simulink model "Bidir3"  (R2024a)
settings: Solver=VariableStepAuto  StartTime=0.0  StopTime=70  MaxStep=0.1  RelTol=1e-3
libraries: simulink x10
settings Model: Creator=SEPTPFNK  LastModifiedBy=skoge
settings DataIOCC: SaveFormat=Array  SaveOutput=off  DSMLogging=off  ReturnWorkspaceOutputs=off  TimeSaveName=t
settings OptimizationCC: ReuseModelBlockBuffer=off
settings RTWCC: GPUComputeCapability=3.5

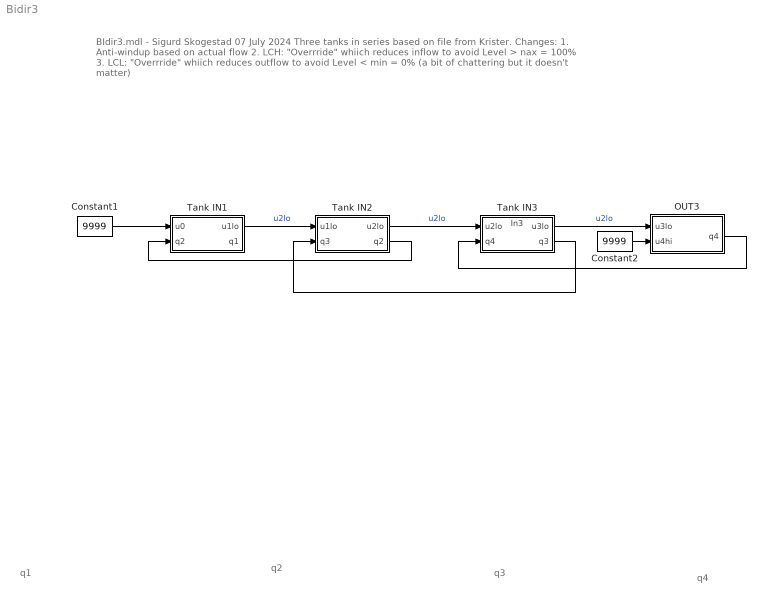
== system Bidir3 ==
  note: q1
  note: BIdir3.mdl - Sigurd Skogestad 07 July 2024
      | Three tanks in series based on file from Krister.
      |
      | Changes: 1. Anti-windup based on actual flow
      | 2. LCH: "Overrride" whiich reduces inflow to avoid Level > nax = 100%
      | 3. LCL: "Overrride" whiich reduces outflow to avoid Level < min = 0% (a bit of chattering but it doesn't matter)
  note: q2
  note: q3
  note: q4
  Constant1 : Constant  Value=9999
  Constant2 : Constant  Value=9999
  OUT3 : Subsystem
  Tank IN1 : Subsystem
  Tank IN2 : Subsystem
  Tank IN3 : Subsystem
      settings: PortSchema="{\"entries\":[{\"content\":{\"sides\":[{\"content\":{\"connectorIds\":[\"In1\",\"In2\"]},\"type\":\"ConnectorPlacement.EquallySpacedRectSide\",\"uuid\":\"ff44d203-131c-4583-b6b4-863d22efac0d\"},{\"content\":{\"connectorIds\":[\"Out1\",\"Out2\"],\"side\":\"RIGHT\"},\"type\":\"ConnectorPlacement.EquallySpacedRectSide\",\"uuid\":\"9e6c79fa-f849-4fea-b46c-ba618541df73\"},{\"content\":{\"connectorIds\":[\"In3\"],\"side\":\"TOP\"},\"type\":\"ConnectorPlacement.EquallySpacedRectSide\",\"uuid\":\"7639274b-f52c-4ba2-a8a4-a7eece00f8f0\"}]},\"type\":\"ConnectorPlacement.EquallySpacedConnector\",\"uuid\":\"d074d2e5-96ed-48a1-ad28-1a607b55dcd0\"}],\"packageUris\":[\"http://schema.mathworks.com/mf0/Connector/R2020b\"],\"version\":\"1.0\"}"
  wires:
  Tank IN1/1(u1lo) -> Tank IN2/1(u1lo)  "u2lo"
  Tank IN2/2(q2) -> Tank IN1/2(q2)
  Constant1/1 -> Tank IN1/1(u0)
  Tank IN2/1(u2lo) -> Tank IN3/1(u2lo)  "u2lo"
  Tank IN3/2(q3) -> Tank IN2/2(q3)
  Tank IN3/1(u3lo) -> OUT3/1(u3lo)  "u2lo"
  Constant2/1 -> OUT3/2(u4hi)
  OUT3/1(q4) -> Tank IN3/2(q4)

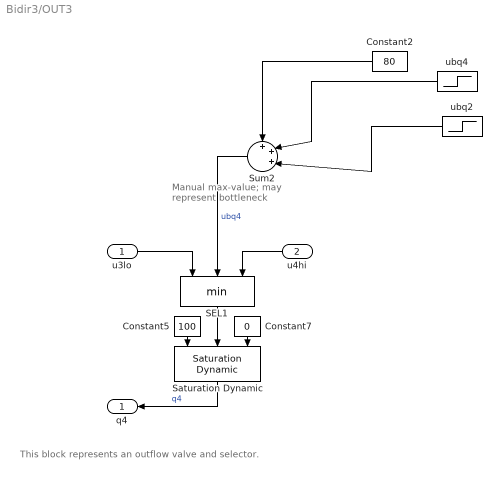
== system Bidir3/OUT3 ==
  note: This block represents an outflow valve and selector.
  note: Manual max-value; may represent bottleneck
  u3lo : Inport
  u4hi : Inport  Port=2
  Constant2 : Constant  Value=80
  Constant5 : Constant  Value=100
  Constant7 : Constant  Value=0
  SEL1 : MinMax  Inputs=3
  Saturation Dynamic : simulink/Discontinuities/Saturation Dynamic  OutMin=[]  OutMax=[]  OutDataTypeStr=Inherit: Same as second input  OutDataType=fixdt(1, 16)  OutScaling=2^-10  DoSatur=off
  Sum2 : Sum  Inputs=+++|
  ubq2 : Step  Time=20  After=-50  SampleTime=0
  ubq4 : Step  Time=10  After=10  SampleTime=0
  q4 : Outport
  wires:
  u3lo/1 -> SEL1/1
  SEL1/1 -> Saturation Dynamic/2
  Constant5/1 -> Saturation Dynamic/1
  Constant7/1 -> Saturation Dynamic/3
  Sum2/1 -> SEL1/2  "ubq4"
  Constant2/1 -> Sum2/1
  ubq2/1 -> Sum2/3
  ubq4/1 -> Sum2/2
  Saturation Dynamic/1 -> q4/1  "q4"
  u4hi/1 -> SEL1/3

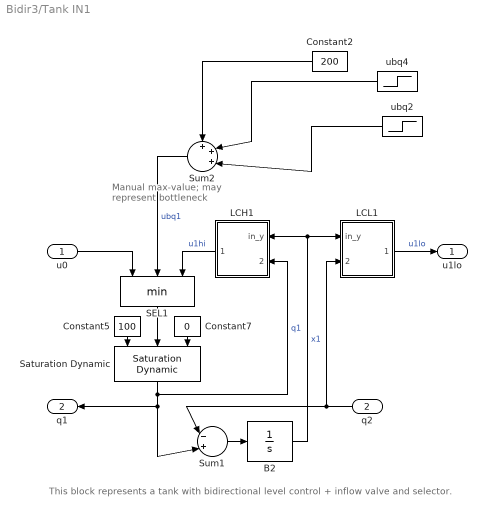
== system Bidir3/Tank IN1 ==
  note: This block represents a tank with bidirectional level control + inflow valve and selector.
  note: Manual max-value; may represent bottleneck
  u0 : Inport
  q2 : Inport  Port=2
  B2 : Integrator  InitialCondition=80  LimitOutput=on  UpperSaturationLimit=200  LowerSaturationLimit=-100
  Constant2 : Constant  Value=200
  Constant5 : Constant  Value=100
  Constant7 : Constant  Value=0
  LCH1 : Subsystem  mask(PID-controller){Kc=1, Ti=4, Tarw=2, r0=80, u0=80, yMin=0, yMax=100, uMin=0, uMax=100}
      mask prompts: Tarw "T_arw"; r0 "Setpoint:"; u0 "Initial output:"
      mask help: PID-controller
      mask Help:
      | <P> PID-controller with beta-factor, limiting, ARW etc </P>
      | 
      | Inputs: <P>
      |  <UL>
      |   1 = r (setpoint) <BR>
      |   2 = y (process value) <BR>
      |   3  = u0 (control signal offset) <BR>
      |  </UL>
      |  </P>
      | Outputs: <P>
      |  <UL>
      |    1 = u (control signal) <BR>
      |    2 = Proportional part  <BR>
      |    3 = Integral part  <BR>
      |    4 = Derivative part  <BR>
      |    5 = raw signal, without ARW  <BR>
      |  </UL>
      |  </P>
      mask Display:
      | disp(['PI' 10 10 10])
      | port_label('input',1,'y')
      | port_label('input',2,'uaw')
      | port_label('output',1,'u')
  LCL1 : Subsystem  mask(PID-controller){Kc=-1, Ti=4, Tarw=2, r0=10, u0=80, yMin=0, yMax=100, uMin=0, uMax=100}
      mask prompts: Tarw "T_arw"; r0 "Setpoint:"; u0 "Initial output:"
      mask help: PID-controller
      mask Help:
      | <P> PID-controller with beta-factor, limiting, ARW etc </P>
      | 
      | Inputs: <P>
      |  <UL>
      |   1 = r (setpoint) <BR>
      |   2 = y (process value) <BR>
      |   3  = u0 (control signal offset) <BR>
      |  </UL>
      |  </P>
      | Outputs: <P>
      |  <UL>
      |    1 = u (control signal) <BR>
      |    2 = Proportional part  <BR>
      |    3 = Integral part  <BR>
      |    4 = Derivative part  <BR>
      |    5 = raw signal, without ARW  <BR>
      |  </UL>
      |  </P>
      mask Display:
      | disp(['PI' 10 10 10])
      | port_label('input',1,'y')
      | port_label('input',2,'uaw')
      | port_label('output',1,'u')
  SEL1 : MinMax  Inputs=3
  Saturation Dynamic : simulink/Discontinuities/Saturation Dynamic  OutMin=[]  OutMax=[]  OutDataTypeStr=Inherit: Same as second input  OutDataType=fixdt(1, 16)  OutScaling=2^-10  DoSatur=off
  Sum1 : Sum  Inputs=|-+|
  Sum2 : Sum  Inputs=+++|
  ubq2 : Step  Time=60  After=-20  SampleTime=0
  ubq4 : Step  Time=40  After=-170  SampleTime=0
  u1lo : Outport
  q1 : Outport  Port=2
  wires:
  B2/1 -> LCL1/1(in_y), LCH1/1(in_y)  "x1"
  u0/1 -> SEL1/1
  SEL1/1 -> Saturation Dynamic/2
  Constant5/1 -> Saturation Dynamic/1
  LCH1/1(out_u) -> SEL1/3  "u1hi"
  Sum1/1 -> B2/1
  Constant7/1 -> Saturation Dynamic/3
  Saturation Dynamic/1 -> Sum1/2, q1/1, LCH1/2(in_yaw)  "q1"
  q2/1 -> LCL1/2(in_yaw), Sum1/1
  Sum2/1 -> SEL1/2  "ubq1"
  Constant2/1 -> Sum2/1
  ubq2/1 -> Sum2/3
  ubq4/1 -> Sum2/2
  LCL1/1(out_u) -> u1lo/1  "u1lo"

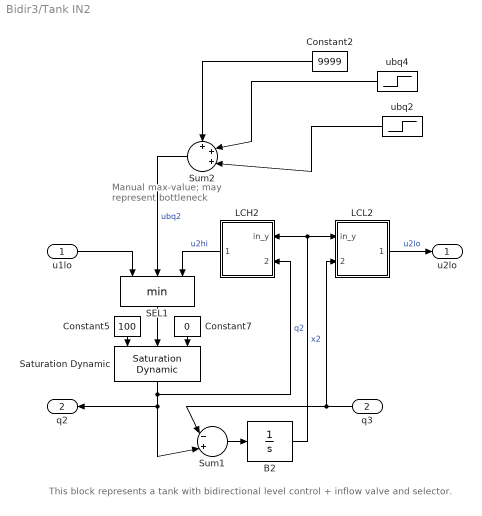
== system Bidir3/Tank IN2 ==
  note: This block represents a tank with bidirectional level control + inflow valve and selector.
  note: Manual max-value; may represent bottleneck
  u1lo : Inport
  q3 : Inport  Port=2
  B2 : Integrator  InitialCondition=80  LimitOutput=on  UpperSaturationLimit=200  LowerSaturationLimit=-100
  Constant2 : Constant  Value=9999
  Constant5 : Constant  Value=100
  Constant7 : Constant  Value=0
  LCH2 : Subsystem  mask(PID-controller){Kc=1, Ti=4, Tarw=2, r0=80, u0=80, yMin=0, yMax=100, uMin=0, uMax=100}
      mask prompts: Tarw "T_arw"; r0 "Setpoint:"; u0 "Initial output:"
      mask help: PID-controller
      mask Help:
      | <P> PID-controller with beta-factor, limiting, ARW etc </P>
      | 
      | Inputs: <P>
      |  <UL>
      |   1 = r (setpoint) <BR>
      |   2 = y (process value) <BR>
      |   3  = u0 (control signal offset) <BR>
      |  </UL>
      |  </P>
      | Outputs: <P>
      |  <UL>
      |    1 = u (control signal) <BR>
      |    2 = Proportional part  <BR>
      |    3 = Integral part  <BR>
      |    4 = Derivative part  <BR>
      |    5 = raw signal, without ARW  <BR>
      |  </UL>
      |  </P>
      mask Display:
      | disp(['PI' 10 10 10])
      | port_label('input',1,'y')
      | port_label('input',2,'uaw')
      | port_label('output',1,'u')
  LCL2 : Subsystem  mask(PID-controller){Kc=-1, Ti=4, Tarw=2, r0=10, u0=80, yMin=0, yMax=100, uMin=0, uMax=100}
      mask prompts: Tarw "T_arw"; r0 "Setpoint:"; u0 "Initial output:"
      mask help: PID-controller
      mask Help:
      | <P> PID-controller with beta-factor, limiting, ARW etc </P>
      | 
      | Inputs: <P>
      |  <UL>
      |   1 = r (setpoint) <BR>
      |   2 = y (process value) <BR>
      |   3  = u0 (control signal offset) <BR>
      |  </UL>
      |  </P>
      | Outputs: <P>
      |  <UL>
      |    1 = u (control signal) <BR>
      |    2 = Proportional part  <BR>
      |    3 = Integral part  <BR>
      |    4 = Derivative part  <BR>
      |    5 = raw signal, without ARW  <BR>
      |  </UL>
      |  </P>
      mask Display:
      | disp(['PI' 10 10 10])
      | port_label('input',1,'y')
      | port_label('input',2,'uaw')
      | port_label('output',1,'u')
  SEL1 : MinMax  Inputs=3
  Saturation Dynamic : simulink/Discontinuities/Saturation Dynamic  OutMin=[]  OutMax=[]  OutDataTypeStr=Inherit: Same as second input  OutDataType=fixdt(1, 16)  OutScaling=2^-10  DoSatur=off
  Sum1 : Sum  Inputs=|-+|
  Sum2 : Sum  Inputs=+++|
  ubq2 : Step  Time=20  After=-20  SampleTime=0
  ubq4 : Step  Time=2  After=20  SampleTime=0
  u2lo : Outport
  q2 : Outport  Port=2
  wires:
  B2/1 -> LCL2/1(in_y), LCH2/1(in_y)  "x2"
  u1lo/1 -> SEL1/1
  SEL1/1 -> Saturation Dynamic/2
  Constant5/1 -> Saturation Dynamic/1
  LCH2/1(out_u) -> SEL1/3  "u2hi"
  Sum1/1 -> B2/1
  Constant7/1 -> Saturation Dynamic/3
  Saturation Dynamic/1 -> LCH2/2(in_yaw), Sum1/2, q2/1  "q2"
  q3/1 -> LCL2/2(in_yaw), Sum1/1
  Sum2/1 -> SEL1/2  "ubq2"
  Constant2/1 -> Sum2/1
  ubq2/1 -> Sum2/3
  ubq4/1 -> Sum2/2
  LCL2/1(out_u) -> u2lo/1  "u2lo"

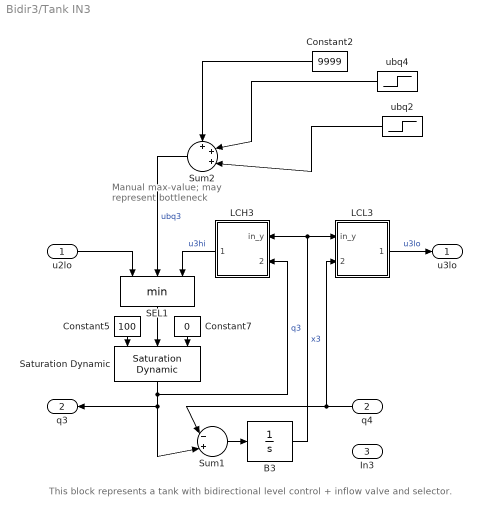
== system Bidir3/Tank IN3 ==
  note: This block represents a tank with bidirectional level control + inflow valve and selector.
  note: Manual max-value; may represent bottleneck
  u2lo : Inport
  q4 : Inport  Port=2
  In3 : Inport  Port=3
  B3 : Integrator  InitialCondition=80  LimitOutput=on  UpperSaturationLimit=200  LowerSaturationLimit=-100
  Constant2 : Constant  Value=9999
  Constant5 : Constant  Value=100
  Constant7 : Constant  Value=0
  LCH3 : Subsystem  mask(PID-controller){Kc=1, Ti=4, Tarw=2, r0=80, u0=80, yMin=0, yMax=100, uMin=0, uMax=100}
      mask prompts: Tarw "T_arw"; r0 "Setpoint:"; u0 "Initial output:"
      mask help: PID-controller
      mask Help:
      | <P> PID-controller with beta-factor, limiting, ARW etc </P>
      | 
      | Inputs: <P>
      |  <UL>
      |   1 = r (setpoint) <BR>
      |   2 = y (process value) <BR>
      |   3  = u0 (control signal offset) <BR>
      |  </UL>
      |  </P>
      | Outputs: <P>
      |  <UL>
      |    1 = u (control signal) <BR>
      |    2 = Proportional part  <BR>
      |    3 = Integral part  <BR>
      |    4 = Derivative part  <BR>
      |    5 = raw signal, without ARW  <BR>
      |  </UL>
      |  </P>
      mask Display:
      | disp(['PI' 10 10 10])
      | port_label('input',1,'y')
      | port_label('input',2,'uaw')
      | port_label('output',1,'u')
  LCL3 : Subsystem  mask(PID-controller){Kc=-1, Ti=4, Tarw=2, r0=10, u0=80, yMin=0, yMax=100, uMin=0, uMax=100}
      mask prompts: Tarw "T_arw"; r0 "Setpoint:"; u0 "Initial output:"
      mask help: PID-controller
      mask Help:
      | <P> PID-controller with beta-factor, limiting, ARW etc </P>
      | 
      | Inputs: <P>
      |  <UL>
      |   1 = r (setpoint) <BR>
      |   2 = y (process value) <BR>
      |   3  = u0 (control signal offset) <BR>
      |  </UL>
      |  </P>
      | Outputs: <P>
      |  <UL>
      |    1 = u (control signal) <BR>
      |    2 = Proportional part  <BR>
      |    3 = Integral part  <BR>
      |    4 = Derivative part  <BR>
      |    5 = raw signal, without ARW  <BR>
      |  </UL>
      |  </P>
      mask Display:
      | disp(['PI' 10 10 10])
      | port_label('input',1,'y')
      | port_label('input',2,'uaw')
      | port_label('output',1,'u')
  SEL1 : MinMax  Inputs=3
  Saturation Dynamic : simulink/Discontinuities/Saturation Dynamic  OutMin=[]  OutMax=[]  OutDataTypeStr=Inherit: Same as second input  OutDataType=fixdt(1, 16)  OutScaling=2^-10  DoSatur=off
  Sum1 : Sum  Inputs=|-+|
  Sum2 : Sum  Inputs=+++|
  ubq2 : Step  Time=20  After=-60  SampleTime=0
  ubq4 : Step  Time=10  After=20  SampleTime=0
  u3lo : Outport
  q3 : Outport  Port=2
  wires:
  B3/1 -> LCH3/1(in_y), LCL3/1(in_y)  "x3"
  u2lo/1 -> SEL1/1
  SEL1/1 -> Saturation Dynamic/2
  Constant5/1 -> Saturation Dynamic/1
  LCH3/1(out_u) -> SEL1/3  "u3hi"
  Sum1/1 -> B3/1
  Constant7/1 -> Saturation Dynamic/3
  Saturation Dynamic/1 -> LCH3/2(in_yaw), Sum1/2, q3/1  "q3"
  q4/1 -> LCL3/2(in_yaw), Sum1/1
  Sum2/1 -> SEL1/2  "ubq3"
  Constant2/1 -> Sum2/1
  ubq2/1 -> Sum2/3
  ubq4/1 -> Sum2/2
  LCL3/1(out_u) -> u3lo/1  "u3lo"

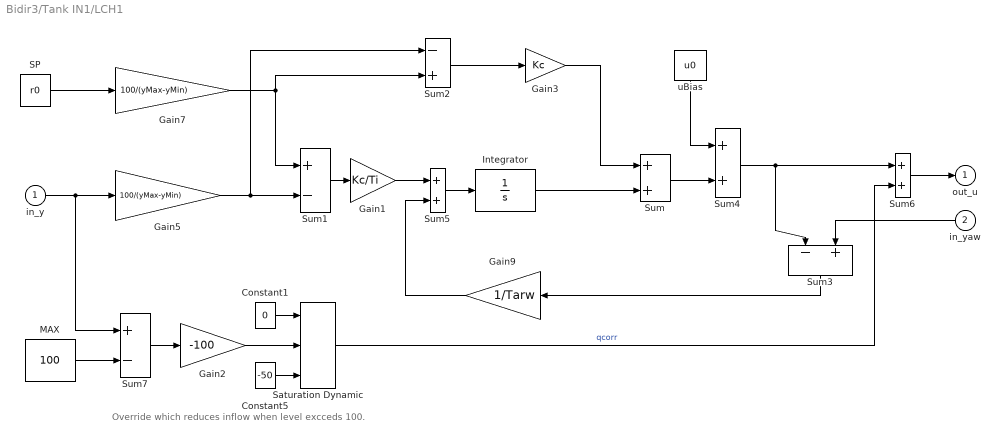
== system Bidir3/Tank IN1/LCH1 ==
  note: Override which reduces inflow when level excceds 100.
  in_y : Inport
  in_yaw : Inport  Port=2
  Constant1 : Constant  Value=0
  Constant5 : Constant  Value=-50
  Gain1 : Gain  Gain=Kc/Ti  SaturateOnIntegerOverflow=on  OutDataTypeStr=Inherit: Same as input  ParamDataTypeStr=Inherit: Same as input
  Gain2 : Gain  Gain=-100  SaturateOnIntegerOverflow=on  OutDataTypeStr=Inherit: Same as input  ParamDataTypeStr=Inherit: Same as input
  Gain3 : Gain  Gain=Kc  SaturateOnIntegerOverflow=on  OutDataTypeStr=Inherit: Same as input  ParamDataTypeStr=Inherit: Same as input
  Gain5 : Gain  Gain=100/(yMax-yMin)  SaturateOnIntegerOverflow=on  OutDataTypeStr=Inherit: Same as input  ParamDataTypeStr=Inherit: Same as input
  Gain7 : Gain  Gain=100/(yMax-yMin)  SaturateOnIntegerOverflow=on  OutDataTypeStr=Inherit: Same as input  ParamDataTypeStr=Inherit: Same as input
  Gain9 : Gain  Gain=1/Tarw  SaturateOnIntegerOverflow=on  OutDataTypeStr=Inherit: Same as input  ParamDataTypeStr=Inherit: Same as input
  Integrator : Integrator
  MAX : Constant  Value=100
  SP : Constant  Value=r0
  Saturation Dynamic : simulink/Discontinuities/Saturation Dynamic  OutMin=[]  OutMax=[]  OutDataTypeStr=Inherit: Same as second input  OutDataType=fixdt(1, 16)  OutScaling=2^-10  DoSatur=off
  Sum{,4..6} (4 alike) : Sum  InputSameDT=on  SaturateOnIntegerOverflow=on  OutDataTypeStr=Inherit: Same as first input
  Sum1 : Sum  Inputs=+-  InputSameDT=on  SaturateOnIntegerOverflow=on  OutDataTypeStr=Inherit: Same as first input
  Sum2 : Sum  Inputs=-+  InputSameDT=on  SaturateOnIntegerOverflow=on  OutDataTypeStr=Inherit: Same as first input
  Sum3 : Sum  Inputs=-+  InputSameDT=on  SaturateOnIntegerOverflow=on  OutDataTypeStr=Inherit: Same as first input
  Sum7 : Sum  Inputs=+-  InputSameDT=on  SaturateOnIntegerOverflow=on  OutDataTypeStr=Inherit: Same as first input
  uBias : Constant  Value=u0
  out_u : Outport  VectorParamsAs1DForOutWhenUnconnected=off
  wires:
  Gain3/1 -> Sum/1
  Sum5/1 -> Integrator/1
  Gain9/1 -> Sum5/2
  Gain1/1 -> Sum5/1
  Sum3/1 -> Gain9/1
  Sum/1 -> Sum4/2
  Sum4/1 -> Sum6/1, Sum3/1
  Gain5/1 -> Sum2/1, Sum1/2
  Sum2/1 -> Gain3/1
  Gain7/1 -> Sum2/2, Sum1/1
  Sum1/1 -> Gain1/1
  in_y/1 -> Sum7/1, Gain5/1
  SP/1 -> Gain7/1
  Integrator/1 -> Sum/2
  uBias/1 -> Sum4/1
  in_yaw/1 -> Sum3/2
  Gain2/1 -> Saturation Dynamic/2
  Constant1/1 -> Saturation Dynamic/1
  Constant5/1 -> Saturation Dynamic/3
  Sum6/1 -> out_u/1
  Saturation Dynamic/1 -> Sum6/2  "qcorr"
  Sum7/1 -> Gain2/1
  MAX/1 -> Sum7/2

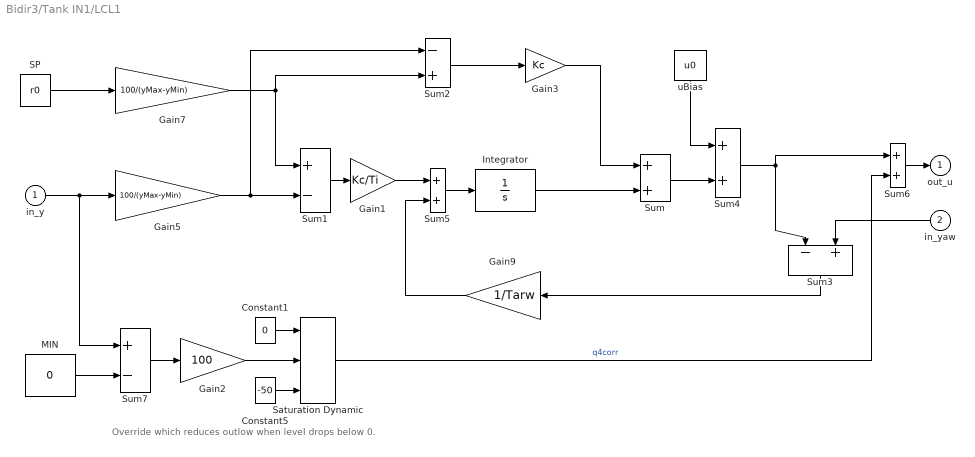
== system Bidir3/Tank IN1/LCL1 ==
  note: Override which reduces outlow when level drops below 0.
  in_y : Inport
  in_yaw : Inport  Port=2
  Constant1 : Constant  Value=0
  Constant5 : Constant  Value=-50
  Gain1 : Gain  Gain=Kc/Ti  SaturateOnIntegerOverflow=on  OutDataTypeStr=Inherit: Same as input  ParamDataTypeStr=Inherit: Same as input
  Gain2 : Gain  Gain=100  SaturateOnIntegerOverflow=on  OutDataTypeStr=Inherit: Same as input  ParamDataTypeStr=Inherit: Same as input
  Gain3 : Gain  Gain=Kc  SaturateOnIntegerOverflow=on  OutDataTypeStr=Inherit: Same as input  ParamDataTypeStr=Inherit: Same as input
  Gain5 : Gain  Gain=100/(yMax-yMin)  SaturateOnIntegerOverflow=on  OutDataTypeStr=Inherit: Same as input  ParamDataTypeStr=Inherit: Same as input
  Gain7 : Gain  Gain=100/(yMax-yMin)  SaturateOnIntegerOverflow=on  OutDataTypeStr=Inherit: Same as input  ParamDataTypeStr=Inherit: Same as input
  Gain9 : Gain  Gain=1/Tarw  SaturateOnIntegerOverflow=on  OutDataTypeStr=Inherit: Same as input  ParamDataTypeStr=Inherit: Same as input
  Integrator : Integrator
  MIN : Constant  Value=0
  SP : Constant  Value=r0
  Saturation Dynamic : simulink/Discontinuities/Saturation Dynamic  OutMin=[]  OutMax=[]  OutDataTypeStr=Inherit: Same as second input  OutDataType=fixdt(1, 16)  OutScaling=2^-10  DoSatur=off
  Sum{,4..6} (4 alike) : Sum  InputSameDT=on  SaturateOnIntegerOverflow=on  OutDataTypeStr=Inherit: Same as first input
  Sum1 : Sum  Inputs=+-  InputSameDT=on  SaturateOnIntegerOverflow=on  OutDataTypeStr=Inherit: Same as first input
  Sum2 : Sum  Inputs=-+  InputSameDT=on  SaturateOnIntegerOverflow=on  OutDataTypeStr=Inherit: Same as first input
  Sum3 : Sum  Inputs=-+  InputSameDT=on  SaturateOnIntegerOverflow=on  OutDataTypeStr=Inherit: Same as first input
  Sum7 : Sum  Inputs=+-  InputSameDT=on  SaturateOnIntegerOverflow=on  OutDataTypeStr=Inherit: Same as first input
  uBias : Constant  Value=u0
  out_u : Outport  VectorParamsAs1DForOutWhenUnconnected=off
  wires:
  Gain3/1 -> Sum/1
  Sum5/1 -> Integrator/1
  Gain9/1 -> Sum5/2
  Gain1/1 -> Sum5/1
  Sum3/1 -> Gain9/1
  Sum/1 -> Sum4/2
  Gain5/1 -> Sum2/1, Sum1/2
  Sum2/1 -> Gain3/1
  Gain7/1 -> Sum2/2, Sum1/1
  Sum1/1 -> Gain1/1
  in_y/1 -> Sum7/1, Gain5/1
  SP/1 -> Gain7/1
  Integrator/1 -> Sum/2
  uBias/1 -> Sum4/1
  in_yaw/1 -> Sum3/2
  Constant5/1 -> Saturation Dynamic/3
  Saturation Dynamic/1 -> Sum6/2  "q4corr"
  MIN/1 -> Sum7/2
  Gain2/1 -> Saturation Dynamic/2
  Sum7/1 -> Gain2/1
  Constant1/1 -> Saturation Dynamic/1
  Sum4/1 -> Sum3/1, Sum6/1
  Sum6/1 -> out_u/1

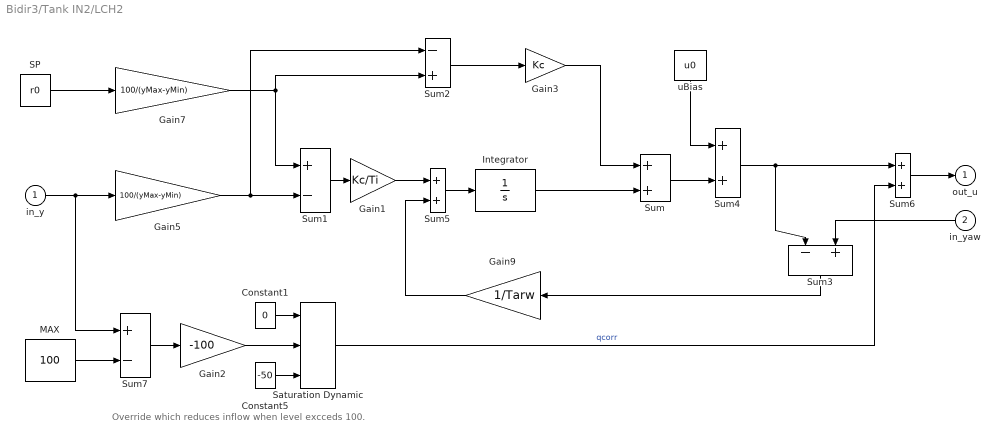
== system Bidir3/Tank IN2/LCH2 ==
  note: Override which reduces inflow when level excceds 100.
  in_y : Inport
  in_yaw : Inport  Port=2
  Constant1 : Constant  Value=0
  Constant5 : Constant  Value=-50
  Gain1 : Gain  Gain=Kc/Ti  SaturateOnIntegerOverflow=on  OutDataTypeStr=Inherit: Same as input  ParamDataTypeStr=Inherit: Same as input
  Gain2 : Gain  Gain=-100  SaturateOnIntegerOverflow=on  OutDataTypeStr=Inherit: Same as input  ParamDataTypeStr=Inherit: Same as input
  Gain3 : Gain  Gain=Kc  SaturateOnIntegerOverflow=on  OutDataTypeStr=Inherit: Same as input  ParamDataTypeStr=Inherit: Same as input
  Gain5 : Gain  Gain=100/(yMax-yMin)  SaturateOnIntegerOverflow=on  OutDataTypeStr=Inherit: Same as input  ParamDataTypeStr=Inherit: Same as input
  Gain7 : Gain  Gain=100/(yMax-yMin)  SaturateOnIntegerOverflow=on  OutDataTypeStr=Inherit: Same as input  ParamDataTypeStr=Inherit: Same as input
  Gain9 : Gain  Gain=1/Tarw  SaturateOnIntegerOverflow=on  OutDataTypeStr=Inherit: Same as input  ParamDataTypeStr=Inherit: Same as input
  Integrator : Integrator
  MAX : Constant  Value=100
  SP : Constant  Value=r0
  Saturation Dynamic : simulink/Discontinuities/Saturation Dynamic  OutMin=[]  OutMax=[]  OutDataTypeStr=Inherit: Same as second input  OutDataType=fixdt(1, 16)  OutScaling=2^-10  DoSatur=off
  Sum{,4..6} (4 alike) : Sum  InputSameDT=on  SaturateOnIntegerOverflow=on  OutDataTypeStr=Inherit: Same as first input
  Sum1 : Sum  Inputs=+-  InputSameDT=on  SaturateOnIntegerOverflow=on  OutDataTypeStr=Inherit: Same as first input
  Sum2 : Sum  Inputs=-+  InputSameDT=on  SaturateOnIntegerOverflow=on  OutDataTypeStr=Inherit: Same as first input
  Sum3 : Sum  Inputs=-+  InputSameDT=on  SaturateOnIntegerOverflow=on  OutDataTypeStr=Inherit: Same as first input
  Sum7 : Sum  Inputs=+-  InputSameDT=on  SaturateOnIntegerOverflow=on  OutDataTypeStr=Inherit: Same as first input
  uBias : Constant  Value=u0
  out_u : Outport  VectorParamsAs1DForOutWhenUnconnected=off
  wires:
  Gain3/1 -> Sum/1
  Sum5/1 -> Integrator/1
  Gain9/1 -> Sum5/2
  Gain1/1 -> Sum5/1
  Sum3/1 -> Gain9/1
  Sum/1 -> Sum4/2
  Sum4/1 -> Sum6/1, Sum3/1
  Gain5/1 -> Sum2/1, Sum1/2
  Sum2/1 -> Gain3/1
  Gain7/1 -> Sum2/2, Sum1/1
  Sum1/1 -> Gain1/1
  in_y/1 -> Sum7/1, Gain5/1
  SP/1 -> Gain7/1
  Integrator/1 -> Sum/2
  uBias/1 -> Sum4/1
  in_yaw/1 -> Sum3/2
  Gain2/1 -> Saturation Dynamic/2
  Constant1/1 -> Saturation Dynamic/1
  Constant5/1 -> Saturation Dynamic/3
  Sum6/1 -> out_u/1
  Saturation Dynamic/1 -> Sum6/2  "qcorr"
  Sum7/1 -> Gain2/1
  MAX/1 -> Sum7/2

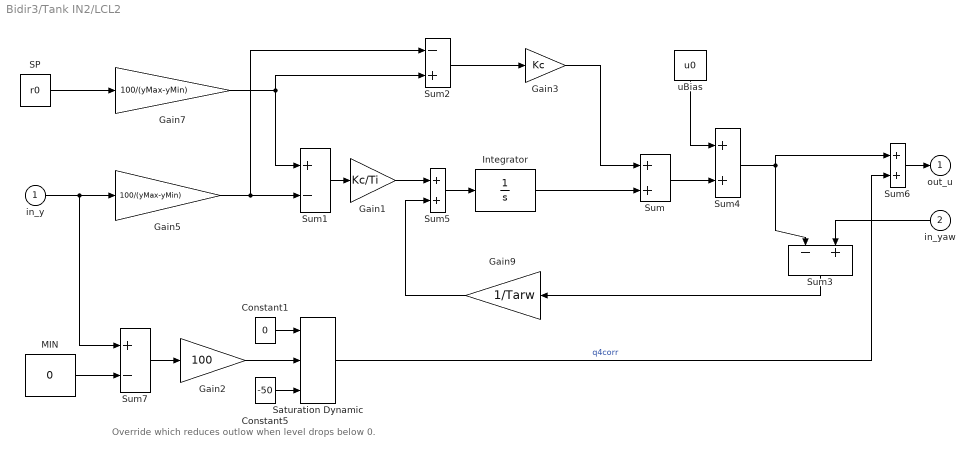
== system Bidir3/Tank IN2/LCL2 ==
  note: Override which reduces outlow when level drops below 0.
  in_y : Inport
  in_yaw : Inport  Port=2
  Constant1 : Constant  Value=0
  Constant5 : Constant  Value=-50
  Gain1 : Gain  Gain=Kc/Ti  SaturateOnIntegerOverflow=on  OutDataTypeStr=Inherit: Same as input  ParamDataTypeStr=Inherit: Same as input
  Gain2 : Gain  Gain=100  SaturateOnIntegerOverflow=on  OutDataTypeStr=Inherit: Same as input  ParamDataTypeStr=Inherit: Same as input
  Gain3 : Gain  Gain=Kc  SaturateOnIntegerOverflow=on  OutDataTypeStr=Inherit: Same as input  ParamDataTypeStr=Inherit: Same as input
  Gain5 : Gain  Gain=100/(yMax-yMin)  SaturateOnIntegerOverflow=on  OutDataTypeStr=Inherit: Same as input  ParamDataTypeStr=Inherit: Same as input
  Gain7 : Gain  Gain=100/(yMax-yMin)  SaturateOnIntegerOverflow=on  OutDataTypeStr=Inherit: Same as input  ParamDataTypeStr=Inherit: Same as input
  Gain9 : Gain  Gain=1/Tarw  SaturateOnIntegerOverflow=on  OutDataTypeStr=Inherit: Same as input  ParamDataTypeStr=Inherit: Same as input
  Integrator : Integrator
  MIN : Constant  Value=0
  SP : Constant  Value=r0
  Saturation Dynamic : simulink/Discontinuities/Saturation Dynamic  OutMin=[]  OutMax=[]  OutDataTypeStr=Inherit: Same as second input  OutDataType=fixdt(1, 16)  OutScaling=2^-10  DoSatur=off
  Sum{,4..6} (4 alike) : Sum  InputSameDT=on  SaturateOnIntegerOverflow=on  OutDataTypeStr=Inherit: Same as first input
  Sum1 : Sum  Inputs=+-  InputSameDT=on  SaturateOnIntegerOverflow=on  OutDataTypeStr=Inherit: Same as first input
  Sum2 : Sum  Inputs=-+  InputSameDT=on  SaturateOnIntegerOverflow=on  OutDataTypeStr=Inherit: Same as first input
  Sum3 : Sum  Inputs=-+  InputSameDT=on  SaturateOnIntegerOverflow=on  OutDataTypeStr=Inherit: Same as first input
  Sum7 : Sum  Inputs=+-  InputSameDT=on  SaturateOnIntegerOverflow=on  OutDataTypeStr=Inherit: Same as first input
  uBias : Constant  Value=u0
  out_u : Outport  VectorParamsAs1DForOutWhenUnconnected=off
  wires:
  Gain3/1 -> Sum/1
  Sum5/1 -> Integrator/1
  Gain9/1 -> Sum5/2
  Gain1/1 -> Sum5/1
  Sum3/1 -> Gain9/1
  Sum/1 -> Sum4/2
  Gain5/1 -> Sum2/1, Sum1/2
  Sum2/1 -> Gain3/1
  Gain7/1 -> Sum2/2, Sum1/1
  Sum1/1 -> Gain1/1
  in_y/1 -> Sum7/1, Gain5/1
  SP/1 -> Gain7/1
  Integrator/1 -> Sum/2
  uBias/1 -> Sum4/1
  in_yaw/1 -> Sum3/2
  Constant5/1 -> Saturation Dynamic/3
  Saturation Dynamic/1 -> Sum6/2  "q4corr"
  MIN/1 -> Sum7/2
  Gain2/1 -> Saturation Dynamic/2
  Sum7/1 -> Gain2/1
  Constant1/1 -> Saturation Dynamic/1
  Sum4/1 -> Sum3/1, Sum6/1
  Sum6/1 -> out_u/1

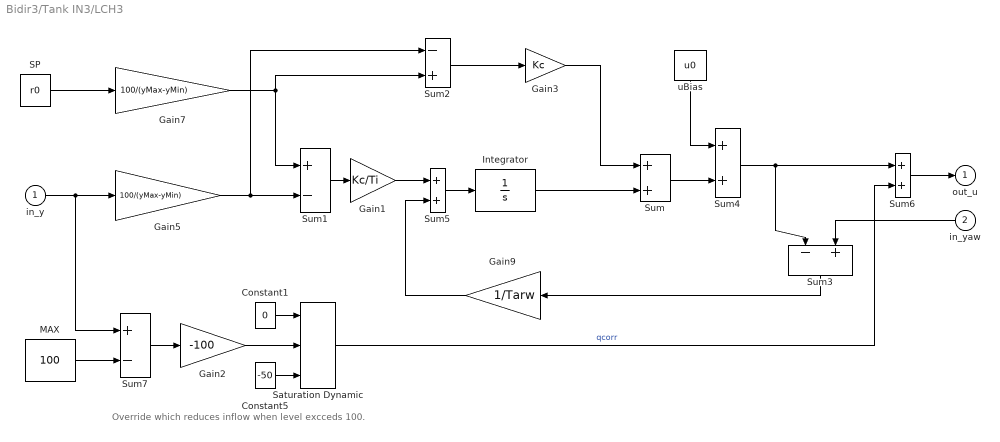
== system Bidir3/Tank IN3/LCH3 ==
  note: Override which reduces inflow when level excceds 100.
  in_y : Inport
  in_yaw : Inport  Port=2
  Constant1 : Constant  Value=0
  Constant5 : Constant  Value=-50
  Gain1 : Gain  Gain=Kc/Ti  SaturateOnIntegerOverflow=on  OutDataTypeStr=Inherit: Same as input  ParamDataTypeStr=Inherit: Same as input
  Gain2 : Gain  Gain=-100  SaturateOnIntegerOverflow=on  OutDataTypeStr=Inherit: Same as input  ParamDataTypeStr=Inherit: Same as input
  Gain3 : Gain  Gain=Kc  SaturateOnIntegerOverflow=on  OutDataTypeStr=Inherit: Same as input  ParamDataTypeStr=Inherit: Same as input
  Gain5 : Gain  Gain=100/(yMax-yMin)  SaturateOnIntegerOverflow=on  OutDataTypeStr=Inherit: Same as input  ParamDataTypeStr=Inherit: Same as input
  Gain7 : Gain  Gain=100/(yMax-yMin)  SaturateOnIntegerOverflow=on  OutDataTypeStr=Inherit: Same as input  ParamDataTypeStr=Inherit: Same as input
  Gain9 : Gain  Gain=1/Tarw  SaturateOnIntegerOverflow=on  OutDataTypeStr=Inherit: Same as input  ParamDataTypeStr=Inherit: Same as input
  Integrator : Integrator
  MAX : Constant  Value=100
  SP : Constant  Value=r0
  Saturation Dynamic : simulink/Discontinuities/Saturation Dynamic  OutMin=[]  OutMax=[]  OutDataTypeStr=Inherit: Same as second input  OutDataType=fixdt(1, 16)  OutScaling=2^-10  DoSatur=off
  Sum{,4..6} (4 alike) : Sum  InputSameDT=on  SaturateOnIntegerOverflow=on  OutDataTypeStr=Inherit: Same as first input
  Sum1 : Sum  Inputs=+-  InputSameDT=on  SaturateOnIntegerOverflow=on  OutDataTypeStr=Inherit: Same as first input
  Sum2 : Sum  Inputs=-+  InputSameDT=on  SaturateOnIntegerOverflow=on  OutDataTypeStr=Inherit: Same as first input
  Sum3 : Sum  Inputs=-+  InputSameDT=on  SaturateOnIntegerOverflow=on  OutDataTypeStr=Inherit: Same as first input
  Sum7 : Sum  Inputs=+-  InputSameDT=on  SaturateOnIntegerOverflow=on  OutDataTypeStr=Inherit: Same as first input
  uBias : Constant  Value=u0
  out_u : Outport  VectorParamsAs1DForOutWhenUnconnected=off
  wires:
  Gain3/1 -> Sum/1
  Sum5/1 -> Integrator/1
  Gain9/1 -> Sum5/2
  Gain1/1 -> Sum5/1
  Sum3/1 -> Gain9/1
  Sum/1 -> Sum4/2
  Sum4/1 -> Sum6/1, Sum3/1
  Gain5/1 -> Sum2/1, Sum1/2
  Sum2/1 -> Gain3/1
  Gain7/1 -> Sum2/2, Sum1/1
  Sum1/1 -> Gain1/1
  in_y/1 -> Sum7/1, Gain5/1
  SP/1 -> Gain7/1
  Integrator/1 -> Sum/2
  uBias/1 -> Sum4/1
  in_yaw/1 -> Sum3/2
  Gain2/1 -> Saturation Dynamic/2
  Constant1/1 -> Saturation Dynamic/1
  Constant5/1 -> Saturation Dynamic/3
  Sum6/1 -> out_u/1
  Saturation Dynamic/1 -> Sum6/2  "qcorr"
  Sum7/1 -> Gain2/1
  MAX/1 -> Sum7/2

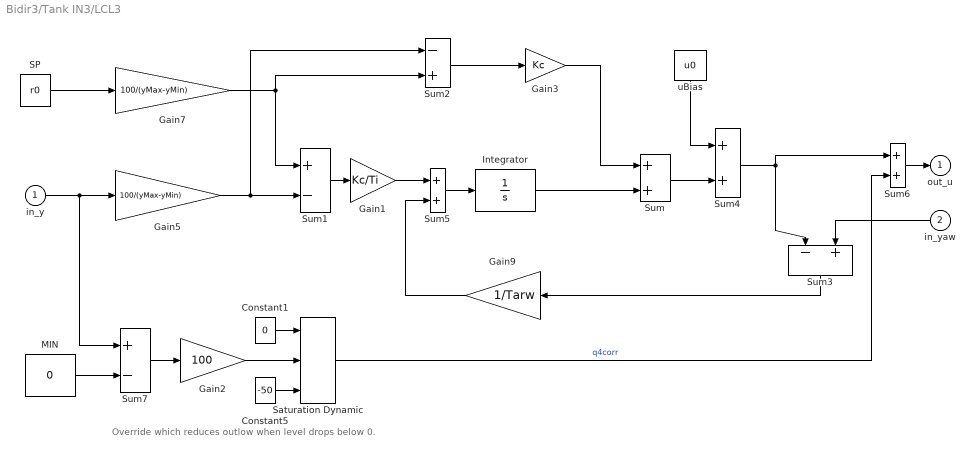
== system Bidir3/Tank IN3/LCL3 ==
  note: Override which reduces outlow when level drops below 0.
  in_y : Inport
  in_yaw : Inport  Port=2
  Constant1 : Constant  Value=0
  Constant5 : Constant  Value=-50
  Gain1 : Gain  Gain=Kc/Ti  SaturateOnIntegerOverflow=on  OutDataTypeStr=Inherit: Same as input  ParamDataTypeStr=Inherit: Same as input
  Gain2 : Gain  Gain=100  SaturateOnIntegerOverflow=on  OutDataTypeStr=Inherit: Same as input  ParamDataTypeStr=Inherit: Same as input
  Gain3 : Gain  Gain=Kc  SaturateOnIntegerOverflow=on  OutDataTypeStr=Inherit: Same as input  ParamDataTypeStr=Inherit: Same as input
  Gain5 : Gain  Gain=100/(yMax-yMin)  SaturateOnIntegerOverflow=on  OutDataTypeStr=Inherit: Same as input  ParamDataTypeStr=Inherit: Same as input
  Gain7 : Gain  Gain=100/(yMax-yMin)  SaturateOnIntegerOverflow=on  OutDataTypeStr=Inherit: Same as input  ParamDataTypeStr=Inherit: Same as input
  Gain9 : Gain  Gain=1/Tarw  SaturateOnIntegerOverflow=on  OutDataTypeStr=Inherit: Same as input  ParamDataTypeStr=Inherit: Same as input
  Integrator : Integrator
  MIN : Constant  Value=0
  SP : Constant  Value=r0
  Saturation Dynamic : simulink/Discontinuities/Saturation Dynamic  OutMin=[]  OutMax=[]  OutDataTypeStr=Inherit: Same as second input  OutDataType=fixdt(1, 16)  OutScaling=2^-10  DoSatur=off
  Sum{,4..6} (4 alike) : Sum  InputSameDT=on  SaturateOnIntegerOverflow=on  OutDataTypeStr=Inherit: Same as first input
  Sum1 : Sum  Inputs=+-  InputSameDT=on  SaturateOnIntegerOverflow=on  OutDataTypeStr=Inherit: Same as first input
  Sum2 : Sum  Inputs=-+  InputSameDT=on  SaturateOnIntegerOverflow=on  OutDataTypeStr=Inherit: Same as first input
  Sum3 : Sum  Inputs=-+  InputSameDT=on  SaturateOnIntegerOverflow=on  OutDataTypeStr=Inherit: Same as first input
  Sum7 : Sum  Inputs=+-  InputSameDT=on  SaturateOnIntegerOverflow=on  OutDataTypeStr=Inherit: Same as first input
  uBias : Constant  Value=u0
  out_u : Outport  VectorParamsAs1DForOutWhenUnconnected=off
  wires:
  Gain3/1 -> Sum/1
  Sum5/1 -> Integrator/1
  Gain9/1 -> Sum5/2
  Gain1/1 -> Sum5/1
  Sum3/1 -> Gain9/1
  Sum/1 -> Sum4/2
  Gain5/1 -> Sum2/1, Sum1/2
  Sum2/1 -> Gain3/1
  Gain7/1 -> Sum2/2, Sum1/1
  Sum1/1 -> Gain1/1
  in_y/1 -> Sum7/1, Gain5/1
  SP/1 -> Gain7/1
  Integrator/1 -> Sum/2
  uBias/1 -> Sum4/1
  in_yaw/1 -> Sum3/2
  Constant5/1 -> Saturation Dynamic/3
  Saturation Dynamic/1 -> Sum6/2  "q4corr"
  MIN/1 -> Sum7/2
  Gain2/1 -> Saturation Dynamic/2
  Sum7/1 -> Gain2/1
  Constant1/1 -> Saturation Dynamic/1
  Sum4/1 -> Sum3/1, Sum6/1
  Sum6/1 -> out_u/1
